simulink model "feedback_plant"  (R2016b)
settings: Solver=ode45  StartTime=0.0  StopTime=10.0  MaxStep=0.1  RelTol=1e-3  EnableMultiTasking=on
settings Model: ModifiedByFormat=The MathWorks Inc.  Creator=The MathWorks, Inc.  LastModifiedBy=The MathWorks Inc.
settings DataIOCC: SaveFormat=Array
settings OptimizationCC: DefaultParameterBehavior=Inlined  ExpressionDepthLimit=2147483647  LifeSpan=1
settings DebuggingCC: UnderspecifiedInitializationDetection=Classic  MergeDetectMultiDrivingBlocksExec=none  SolverPrmCheckMsg=warning  FcnCallInpInsideContextMsg=warning  AllowSymbolicDim=off  StateNameClashWarn=warning  SFUnexpectedBacktrackingDiag=warning  SFNoUnconditionalDefaultTransitionDiag=warning  SFExecutionAtInitializationDiag=none
settings HardwareCC: ProdBitPerPointer=32  ProdBitPerSizeT=32  ProdBitPerPtrDiffT=32  ProdLargestAtomicFloat=None  ProdIntDivRoundTo=Undefined  ProdEndianess=Unspecified  ProdWordSize=32  ProdHWDeviceType=32-bit Generic
settings ModelReferenceCC: PropagateSignalLabelsOutOfModel=off
settings GRTTargetCC: TargetLangStandard=C89/C90 (ANSI)  GeneratePreprocessorConditionals=Disable all  CombineOutputUpdateFcns=off  GRTInterface=on
settings ConfigComp: CovMetricSettings=dw  CovHtmlReporting=on  CovSaveCumulativeToWorkspaceVar=on  CovSaveSingleToWorkspaceVar=on  CovExternalEMLEnable=off  CovSFcnEnable=off

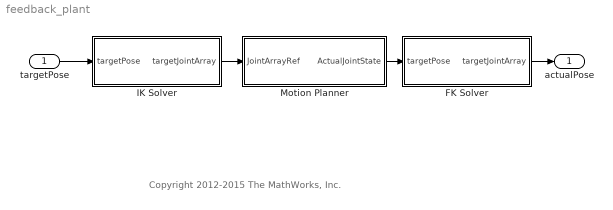
== system feedback_plant ==
  note: Copyright 2012-2015 The MathWorks, Inc.
  targetPose : Inport
  FK Solver : Subsystem
  IK Solver : Subsystem
  Motion Planner : Subsystem
  actualPose : Outport
  wires:
  targetPose/1 -> IK Solver/1(targetPose)
  IK Solver/1(targetJointArray) -> Motion Planner/1(JointArrayRef)
  Motion Planner/1(ActualJointState) -> FK Solver/1(targetPose)
  FK Solver/1(targetJointArray) -> actualPose/1

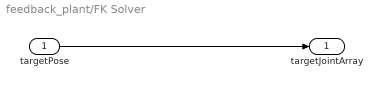
== system feedback_plant/FK Solver ==
  targetPose : Inport  PortDimensions=6
  targetJointArray : Outport
  wires:
  targetPose/1 -> targetJointArray/1

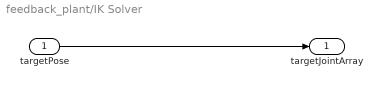
== system feedback_plant/IK Solver ==
  targetPose : Inport  PortDimensions=6
  targetJointArray : Outport
  wires:
  targetPose/1 -> targetJointArray/1

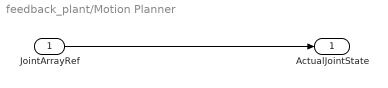
== system feedback_plant/Motion Planner ==
  JointArrayRef : Inport  PortDimensions=6
  ActualJointState : Outport
  wires:
  JointArrayRef/1 -> ActualJointState/1
